simulink model "drift_ex1"  (Simulink 5.0)
settings: Solver=ode45  StartTime=0.0  StopTime=1999  RelTol=1e-3
settings Model: Creator=aruntangirala  LastModifiedBy=aruntangirala  ExtModeAutoUpdateStatusClock=off

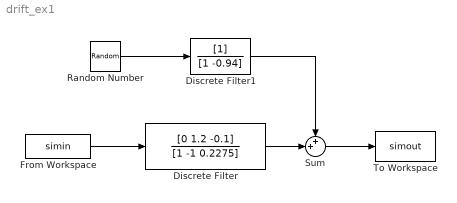
== system drift_ex1 ==
  Discrete Filter : DiscreteFilter  Numerator=[0 1.2 -0.1]  Denominator=[1 -1 0.2275]
  Discrete Filter1 : DiscreteFilter  Denominator=[1 -0.94]
  From Workspace : FromWorkspace  VariableName=simin  SampleTime=0
  Random Number : RandomNumber  Variance=0.1  SampleTime=1
  Sum : Sum  Inputs=++|  SaturateOnIntegerOverflow=on
  To Workspace : ToWorkspace  VariableName=simout  SampleTime=-1  SaveFormat=Array
  wires:
  From Workspace/1 -> Discrete Filter/1
  Random Number/1 -> Discrete Filter1/1
  Discrete Filter1/1 -> Sum/1
  Discrete Filter/1 -> Sum/2
  Sum/1 -> To Workspace/1
